simulink model "untitled3"  (R2024a)
settings: Solver=VariableStepAuto  StartTime=0.0  StopTime=0.0001  MaxStep=0.000000001  MinStep=0.0000000001  RelTol=1e-3
undefined symbols (not defined in the file): A, B, C, D
settings Model: Creator=Perij  LastModifiedBy=Perij
settings SolverCC: InitialStep=0.0000000001

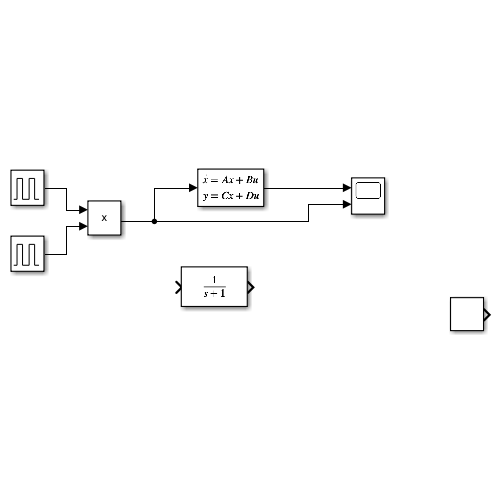
[thumbnail: Simulink's stored preview of the top-level diagram]
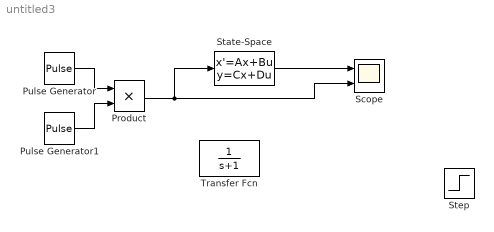
== system untitled3 ==
  Product : Product
  Pulse Generator : DiscretePulseGenerator  PulseType=Time based  Amplitude=330  Period=0.0000043  PulseWidth=50
  Pulse Generator1 : DiscretePulseGenerator  PulseType=Time based  Period=0.0001  PulseWidth=50
  Scope : Scope  NumInputPorts=2
  State-Space : StateSpace  A=A  B=B  C=C  D=D  InitialCondition=0  ParameterTunability=Unconstrained
  Step : Step  Time=0.0001  Before=1  After=0  SampleTime=0
  Transfer Fcn : TransferFcn  Denominator=[1 1]
  wires:
  State-Space/1 -> Scope/1
  Pulse Generator/1 -> Product/1
  Product/1 -> Scope/2, State-Space/1
  Pulse Generator1/1 -> Product/2
